simulink model "project_model_part5_covert_attack"  (R2020a)
settings: Solver=VariableStepAuto  StartTime=0.0  StopTime=50  RelTol=1e-3
undefined symbols (not defined in the file or in its folder): Discrete, Time
libraries: ctrlSharedLib x1
settings Model: Creator=Admin  LastModifiedBy=Shreya
settings DataIOCC: ReturnWorkspaceOutputs=off
settings DebuggingCC: ArithmeticOperatorsInVariantConditions=warning
settings SFSimCC: SimUseLocalCustomCode=off  CustomCodeUndefinedFunction=UseInterfaceOnly
settings RTWCC: RTWUseLocalCustomCode=off

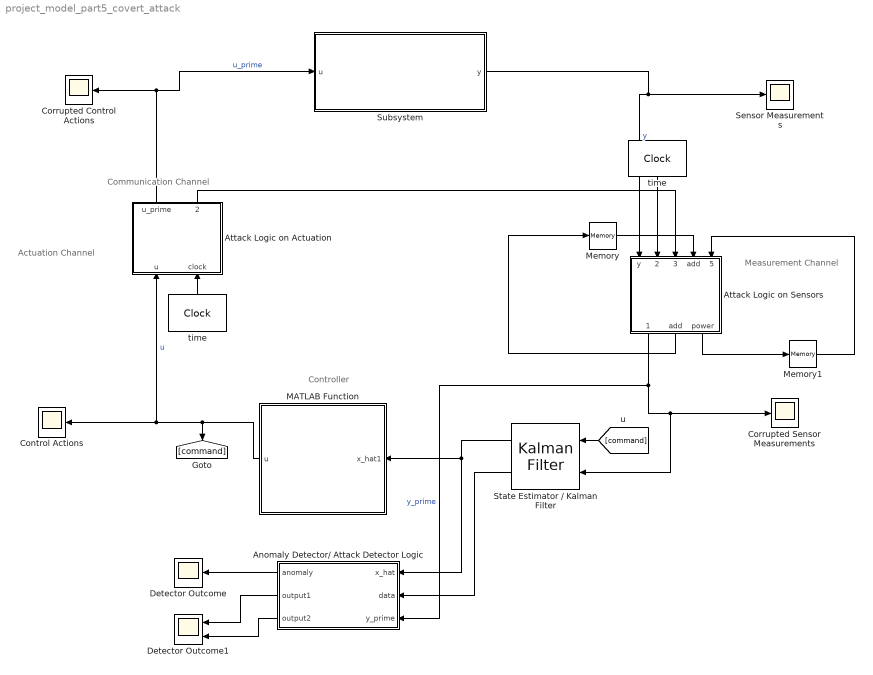
== system project_model_part5_covert_attack ==
  note: Controller
  note: Communication Channel
  note: Measurement Channel
  note: Actuation Channel
  Anomaly Detector/ Attack Detector Logic : MATLAB Function  TreatAsAtomicUnit=on
  Attack Logic on Actuation : MATLAB Function  TreatAsAtomicUnit=on
  Attack Logic on Sensors : MATLAB Function  TreatAsAtomicUnit=on
  Control Actions : Scope
  Corrupted Control Actions : Scope
  Corrupted Sensor Measurements : Scope
  Detector Outcome : Scope
  Detector Outcome1 : Scope  NumInputPorts=2
  MATLAB Function : MATLAB Function  TreatAsAtomicUnit=on
  Memory : Memory  InitialCondition=[0,0,0]  InheritSampleTime=on
  Memory1 : Memory  InheritSampleTime=on
  "Sensor Measurements " : Scope
  State Estimator / Kalman Filter : ctrlSharedLib/Kalman Filter  TimeDomain=Discrete-Time  UseCurrentEstimator=on  ModelSource=Individual A, B, C, D matrices  ModelSourceVariable=sys  A="[1.0000    0.0001   -0.0010;0.5747    1.0000   -0.0003;0.0162    0.0000    1.0000]"  B="[0.1   -0.2; -0.0536    0.0332;0.1955   -0.5294];"  C=[1 0 0;0 1 0]  D=[0 0;0 0]  NumberOfStates=2  NumberOfInputs=2  NumberOfOutputs=2  InitialEstimateSource=Dialog  X0=[0;0;0]  P0=10  UseK=off  UseGH=off  NumberOfProcessNoiseInputs=2  G=1  TimeInvariantG=on  H=0  TimeInvariantH=on  Q=0.00001*eye(3)  TimeInvariantQ=on  R=0.00008*eye(2)  TimeInvariantR=on  N=0  TimeInvariantN=on  AddInputPort=on  AddEnablePort=off  OutputEstimatedY=off  OutputP=on  Ts=-1
  Subsystem : Subsystem
  time : DigitalClock  SampleTime=0.1
  "time " : DigitalClock  SampleTime=0.1
  wires:
  "time "/1 -> Attack Logic on Sensors/2(clock)
  Attack Logic on Sensors/1(y_prime) -> Anomaly Detector/ Attack Detector Logic/3(y_prime), Corrupted Sensor Measurements/1, State Estimator / Kalman Filter/2  "y_prime"
  MATLAB Function/1(u) -> Control Actions/1, Attack Logic on Actuation/1(u), [command]  "u"
  time/1 -> Attack Logic on Actuation/2(clock)
  Attack Logic on Actuation/1(u_prime) -> Subsystem/1(u), Corrupted Control Actions/1  "u_prime"
  [command] -> State Estimator / Kalman Filter/1
  Subsystem/1(y) -> "Sensor Measurements "/1, Attack Logic on Sensors/1(y)  "y"
  State Estimator / Kalman Filter/1 -> MATLAB Function/1(x_hat1), Anomaly Detector/ Attack Detector Logic/1(x_hat)
  Attack Logic on Actuation/2(attack_vector) -> Attack Logic on Sensors/3(attack_vector)
  Attack Logic on Sensors/2(add) -> Memory/1
  Memory/1 -> Attack Logic on Sensors/4("add ")
  Attack Logic on Sensors/3(power) -> Memory1/1
  Memory1/1 -> Attack Logic on Sensors/5("power ")
  State Estimator / Kalman Filter/2 -> Anomaly Detector/ Attack Detector Logic/2(data)
  Anomaly Detector/ Attack Detector Logic/1(anomaly) -> Detector Outcome/1
  Anomaly Detector/ Attack Detector Logic/2(output1) -> Detector Outcome1/1
  Anomaly Detector/ Attack Detector Logic/3(output2) -> Detector Outcome1/2

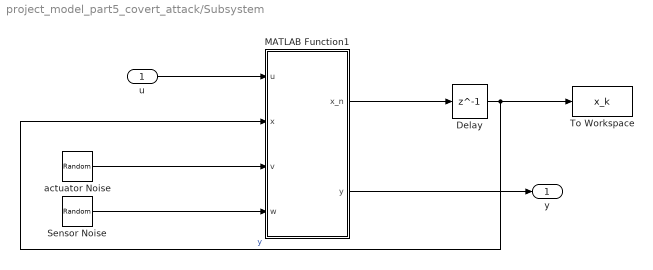
== system project_model_part5_covert_attack/Subsystem ==
  u : Inport
  Delay : Delay  DelayLength=1  InitialCondition=[0 0.1 0.2]
  MATLAB Function1 : MATLAB Function  TreatAsAtomicUnit=on
  Sensor Noise : RandomNumber  Mean=[0 0]  Variance=[0.00008 0.00008]  Seed=[randi(100) randi(100)]
  To Workspace : ToWorkspace  VariableName=x_k  SaveFormat=Timeseries  SampleTime=-1
  actuator Noise : RandomNumber  Mean=[0 0 0]  Variance=[0.00001 0.00001 0.00001]  Seed=[randi(100) randi(100) randi(100)]
  y : Outport  VectorParamsAs1DForOutWhenUnconnected=off
  wires:
  u/1 -> MATLAB Function1/1(u)
  MATLAB Function1/1(x_n) -> Delay/1
  MATLAB Function1/2(y) -> y/1
  Sensor Noise/1 -> MATLAB Function1/4(w)
  actuator Noise/1 -> MATLAB Function1/3(v)
  Delay/1 -> To Workspace/1, MATLAB Function1/2(x)  "y"

== matlab function project_model_part5_covert_attack/Attack Logic on Sensors ==
  data: y input; y_prime output; clock input; attack_vector input; add input; power input; add output; power output
function [y_prime,add,power] = fcn(y,clock,attack_vector,add ,power)
% this function should contain the attacker action on the sensor
% measurements
%attack logic on sensor measurement. Here attacker know plant model(value of
%matrix A,B,C)
y_prime = y;
A = [1.0000 ,0.0001 ,-0.0010;0.5747 ,1.0000 ,-0.0003;0.0162 ,0.0000 ,1.0000];
B = [0.1 ,-0.2; -0.0536 ,0.0332;0.1955 ,-0.5294];
C = [1 ,0 ,0;0 ,1 ,0];
if (clock >= 40) && (clock < 50)
       add = add + ((A^power) * B * attack_vector);
       C_mul_add = C * add;
       y_prime = y - (C_mul_add);
       power = power + 1;
end
end

== matlab function project_model_part5_covert_attack/MATLAB Function ==
  data: x_hat1 input; u output
function u  = Controller(x_hat1)
%two tanks model 
    

%controller gain
K =[17.1291   -1.1789   -6.5335; -0.1248   -2.9385   -2.5082];
u=-K*(x_hat1);

== matlab function project_model_part5_covert_attack/Attack Logic on Actuation ==
  data: u input; u_prime output; clock input; attack_vector output
function [u_prime ,attack_vector] = fcn(u,clock)
% this function should contain the attacker action on the control inputs

% u_a defind as attack vector on actuation channel
attack_vector = transpose([-0.18 ,-0.18]);
if 0 <= clock && clock < 40
    u_a = transpose([0,0]);
elseif clock >= 40 && clock < 50
    u_a = attack_vector;
else 
    u_a = transpose([0,0]);
end
u_prime = u + u_a;
end

== matlab function project_model_part5_covert_attack/Anomaly Detector// Attack Detector Logic ==
  data: x_hat input; anomaly output; output1 output; output2 output; data input; y_prime input
function [anomaly, output1, output2] = Detector(x_hat, data ,y_prime)
% this function should contain the detection strategy

% for the chi square detector "z" should be the name of detection signal and
% "tau" the name of threshold
% Chi-square detection algoritm
C = [1 0 0; 0 1 0];
R = 0.00008*eye(2);
P = data;
sigma = (C * P * (transpose(C))) + R;
r = y_prime - (C * x_hat);
% Detection signal
z = transpose(r) * (inv(sigma) * r);
alpha = 0.01;
v = size(r);
% Threshold
tau = chi2inv(1-alpha , v);
if z <= tau
    alarm = 'NO';
    anomaly = 0;
else
    alarm = 'YES';
    anomaly = 1;
end
output1 = z;
output2 = tau;
end

== matlab function project_model_part5_covert_attack/Subsystem/MATLAB Function1 ==
  data: x_n output; u input; y output; x input; v input; w input
function [x_n, y] = fcn(u, x, v, w)

A=[1.0000    0.0001   -0.0010;0.5747    1.0000   -0.0003;0.0162    0.0000    1.0000];
B = [0.1   -0.2; -0.0536    0.0332;0.1955   -0.5294];

C=[1 0 0;0 1 0];
D=[0 0;0 0];


x_n = A*x + B*u + v;
y = C*x + D*u + w;
